simulink model "robot_LAB__1_3"  (R2024b)
settings: Solver=VariableStepAuto  StartTime=0.0  StopTime=total_time  RelTol=1e-3
values from neighbouring files (symbols this model uses):
  d_nom = 0.165    [MAIN_ROBOT.m]    (also in init_LAB__2.m)
  mode = 2    [MAIN_ROBOT.m]    (also in init_LAB__2.m)
  omega_trj = 2*pi    (= 6.28318530718)    [MAIN_ROBOT.m]    (also in init_LAB__2.m)
  R = 0.4    [MAIN_ROBOT.m]    (also in init_LAB__2.m)
  r_nom = 0.03    [MAIN_ROBOT.m]    (also in init_LAB__2.m)
  Ta = 1    [MAIN_ROBOT.m]    (also in init_LAB__2.m)
  Tc = 30    [MAIN_ROBOT.m]    (also in init_LAB__2.m)
  total_time = 40    [MAIN_ROBOT.m]    (also in init_LAB__2.m = 35)
libraries: dspsigops x2
settings Model: Creator=leontecosm  LastModifiedBy=cosmi

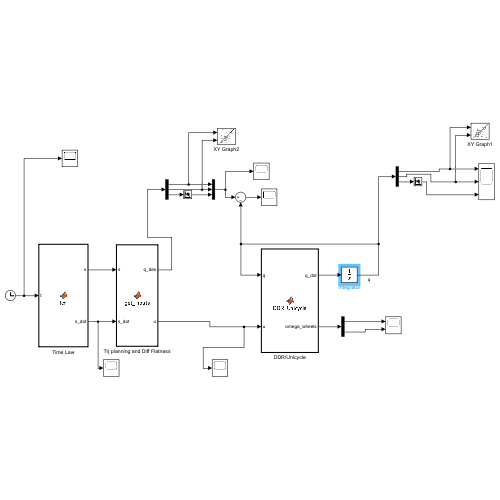
[thumbnail: Simulink's stored preview of the top-level diagram]
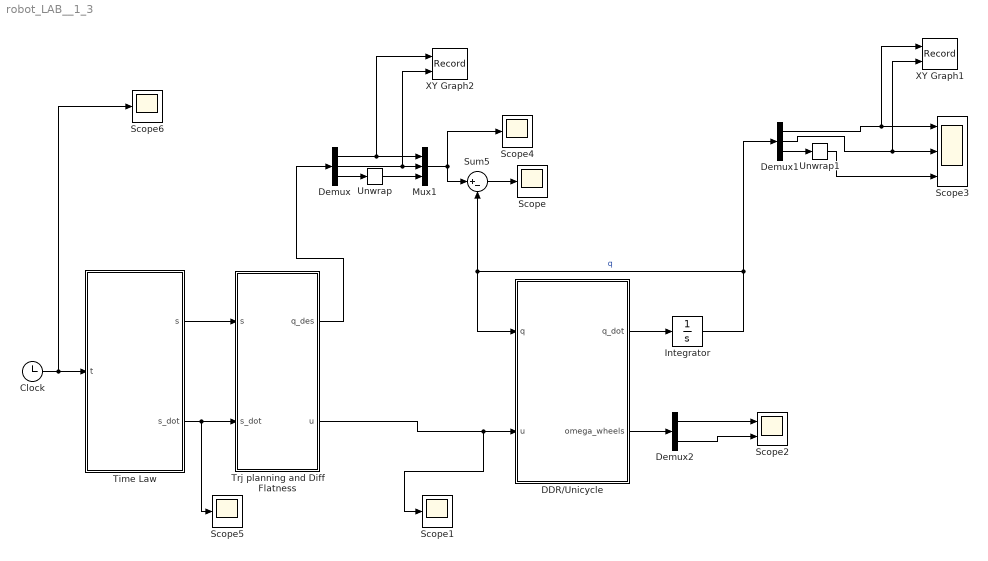
== system robot_LAB__1_3 ==
  Clock : Clock
      settings: Decimation=1/Ts
  DDR/Unicycle : MATLAB Function  TreatAsAtomicUnit=on
  Demux : Demux  Outputs=3
  Demux1 : Demux  Outputs=3
  Demux2 : Demux  Outputs=2
  Integrator : Integrator  InitialCondition=[0,0,pi/7]'
  Mux1 : Mux  Inputs=3
  Scope{,1,4..6} (5 alike) : Scope
  Scope2 : Scope  NumInputPorts=2
  Scope3 : Scope  NumInputPorts=3
  Sum5 : Sum  Inputs=|+-
  Time Law : MATLAB Function  TreatAsAtomicUnit=on
  Trj planning and Diff Flatness : MATLAB Function  TreatAsAtomicUnit=on
  Unwrap : dspsigops/Unwrap  tol=pi  InputProcessing=Columns as channels (frame based)  running=off
  Unwrap1 : dspsigops/Unwrap  tol=pi  InputProcessing=Columns as channels (frame based)  running=off
  XY Graph1 : Record  FileSettingsInternal="{\"entries\":[{\"content\":{\"excelSettings\":{\"content\":{},\"type\":\"Streamout.ExcelSettings\"}},\"type\":\"Streamout.FileSettingStorage\",\"uuid\":\"\"}],\"packageUris\":[\"http:\\/\\/schema.mathworks.com\\/mf0\\/streamout_blocks\\/R2020a\"],\"version\":\"1.0\"}"  Layout=[1 1]  SignalsInternal="{\"entries\":[{\"content\":{\"signals\":[{\"content\":{\"blockPath\":[],\"dimensions\":[1,1],\"domain\":\"\",\"lineColor\":\"#a2142f\",\"plots\":[ 1 ],\"port\":1,\"sid\":[\"\"],\"signalID\":1,\"signalName\":\"Demux1:1\"},\"type\":\"RecordBlkView.Signal\",\"uuid\":\"\"},{\"content\":{\"blockPath\":[],\"dimensions\":[1,1],\"domain\":\"\",\"lineColor\":\"#139fff\",\"plots\":[ 1 ],\"port\":2,\"sid\":[\"\"],\"signalID\":2,\"signalName\":\"Demux1:2\"},\"type\":\"RecordBlkView.Signal\",\"uuid\":\"\"}]},\"type\":\"RecordBlkView.InputSignals\",\"uuid\":\"\"}],\"packageUris\":[\"http:\\/\\/schema.mathworks.com\\/mf0\\/streamout_blocks\\/R2020a\"],\"version\":\"1.0\"}"  VisualizationBindings="{\"xyplotplugin\":{\"info\":[{\"series\":[{\"bindingParametersList\":[{\"parameter\":\"X-Axis\",\"signalID\":1,\"signalName\":\"Demux1:1\"},{\"parameter\":\"Y-Axis\",\"signalID\":2,\"signalName\":\"Demux1:2\"}],\"seriesID\":0}],\"subplotID\":1}]}}"  CompatibilityTag=XY
  XY Graph2 : Record  FileSettingsInternal="{\"entries\":[{\"content\":{\"excelSettings\":{\"content\":{},\"type\":\"Streamout.ExcelSettings\"}},\"type\":\"Streamout.FileSettingStorage\",\"uuid\":\"\"}],\"packageUris\":[\"http:\\/\\/schema.mathworks.com\\/mf0\\/streamout_blocks\\/R2020a\"],\"version\":\"1.0\"}"  Layout=[1 1]  SignalsInternal="{\"entries\":[{\"content\":{\"signals\":[{\"content\":{\"blockPath\":[],\"dimensions\":[1,1],\"domain\":\"\",\"lineColor\":\"#a2142f\",\"plots\":[ 1 ],\"port\":1,\"sid\":[\"\"],\"signalID\":1,\"signalName\":\"Demux:1\"},\"type\":\"RecordBlkView.Signal\",\"uuid\":\"\"},{\"content\":{\"blockPath\":[],\"dimensions\":[1,1],\"domain\":\"\",\"lineColor\":\"#139fff\",\"plots\":[ 1 ],\"port\":2,\"sid\":[\"\"],\"signalID\":2,\"signalName\":\"Demux:2\"},\"type\":\"RecordBlkView.Signal\",\"uuid\":\"\"}]},\"type\":\"RecordBlkView.InputSignals\",\"uuid\":\"\"}],\"packageUris\":[\"http:\\/\\/schema.mathworks.com\\/mf0\\/streamout_blocks\\/R2020a\"],\"version\":\"1.0\"}"  VisualizationBindings="{\"xyplotplugin\":{\"info\":[{\"series\":[{\"bindingParametersList\":[{\"parameter\":\"X-Axis\",\"signalID\":1,\"signalName\":\"Demux:1\"},{\"parameter\":\"Y-Axis\",\"signalID\":2,\"signalName\":\"Demux:2\"}],\"seriesID\":0}],\"subplotID\":1}]}}"  CompatibilityTag=XY
  wires:
  Demux/3 -> Unwrap/1
  Integrator/1 -> Demux1/1, Sum5/2, DDR/Unicycle/1(q)  "q"
  DDR/Unicycle/2(omega_wheels) -> Demux2/1
  Sum5/1 -> Scope/1
  DDR/Unicycle/1(q_dot) -> Integrator/1
  Unwrap/1 -> Mux1/3
  Mux1/1 -> Sum5/1, Scope4/1
  Demux1/3 -> Unwrap1/1
  Trj planning and Diff Flatness/1(q_des) -> Demux/1
  Trj planning and Diff Flatness/2(u) -> Scope1/1, DDR/Unicycle/2(u)
  Demux2/1 -> Scope2/1
  Demux2/2 -> Scope2/2
  Unwrap1/1 -> Scope3/3
  Time Law/1(s) -> Trj planning and Diff Flatness/1(s)
  Time Law/2(s_dot) -> Scope5/1, Trj planning and Diff Flatness/2(s_dot)
  Clock/1 -> Scope6/1, Time Law/1(t)
  Demux1/2 -> XY Graph1/2, Scope3/2
  Demux1/1 -> XY Graph1/1, Scope3/1
  Demux/2 -> XY Graph2/2, Mux1/2
  Demux/1 -> XY Graph2/1, Mux1/1

== matlab function robot_LAB__1_3/Time Law ==
  data: t input; s output; s_dot output; total_time parameter; mode parameter; Ta parameter; Tc parameter
function [s, s_dot] = fcn(t,total_time, mode,Ta, Tc)
s=0;
s_dot=0;

if mode==1%if mode =1 costasnt time law else trapezoidal
    s_dot = 1/total_time;
    s=t/total_time;
else
   

    Vc=1/(Ta+Tc);% velocità costante
    a=Vc/Ta;% acceleration
    
    switch 1 %formula on the slide
        case t<Ta
            s_dot=a*t;
            s=(a*(t^2))/2;

        case (t>=Ta)&&(t<(Tc+Ta))
            s_dot=Vc;
            s=(a*(Ta^2))/2+Vc*(t-Ta);

        case (t>=(Tc+Ta))&&(t<(Tc+2*Ta))
            s_dot=Vc-a*(t-Ta-Tc);
            s=(a*(Ta^2))/2+Vc*Tc+Vc*(t-Ta-Tc)-a*(t-Ta-Tc)^2/2;

        case t>=(Tc+2*Ta)
            s_dot=0;
            s=1;
    end

end

== matlab function robot_LAB__1_3/DDR//Unicycle ==
  data: q input; u input; q_dot output; omega_wheels output; d_nom parameter; r_nom parameter
function [q_dot, omega_wheels] = DDR_Unicycle(q, u, d_nom, r_nom)
v = u(1);
omega = u(2);

q_dot = [cos(q(3))*v; sin(q(3))*v; omega];

%evaluation of speed wheels
omega_L = (2*v - d_nom*omega) / (2*r_nom);
omega_R = (2*v + d_nom*omega) / (2*r_nom);
omega_wheels=[omega_R; omega_L];

== matlab function robot_LAB__1_3/Trj planning and Diff Flatness ==
  data: q_des output; u output; R parameter; omega_trj parameter; s input; s_dot input
function [q_des, u] = get_inputs(R,omega_trj, s, s_dot)

x=R*sin(2*omega_trj.*s);
y=R*sin(omega_trj.*s);

x_dot = R*2*omega_trj*cos(2*omega_trj.*s);
y_dot = R*omega_trj*cos(omega_trj.*s);

x_ddot = R*4*omega_trj*omega_trj*(-sin(2*omega_trj.*s));
y_ddot = R*omega_trj*omega_trj*(-sin(omega_trj.*s));

theta = atan2(y_dot,x_dot);

%   v
v = s_dot*sqrt(y_dot^2 + x_dot^2);

%   omega
w = s_dot*(x_dot*y_ddot - y_dot*x_ddot)/(y_dot^2 + x_dot^2);
    
q_des = [x; y; theta];
u = [v; w];
